simulink model "robust_tracking_LQR"  (R2024b)
settings: Solver=VariableStepAuto  StartTime=0.0  StopTime=10.0  RelTol=1e-3
values from neighbouring files (symbols this model uses):
  current2Torque = mot.Kt    [simulation.m]
  denDriv = [Tdrv 1]    [simulation.m]
  denElect = [mot.L Req]    [simulation.m]
  denMech = [J_eq B_eq]    [simulation.m]
  Ki = Kp / Ti    [PID_SCRIPT.m]    (also in PID_controller.m; simulation.m)
  numDriv = [kdrv]    [simulation.m]
  numElect = [1]    [simulation.m]
  numMech = [1]    [simulation.m]
  speed2Voltage = mot.Ke    [simulation.m]
  Tau = 9.4e-3    (= 0.0094)    [StateSpaceScript.m]
undefined symbols (not defined in the file or in its folder): daq, degs2rpm, denBeam, denHPF, drv, gbox, kappa, Nu, numBeam, numHPF, Nx, rads2rpm, rpm2rads, sens, ssc_LQR_aug
settings Model: Creator=Davide Pillon  LastModifiedBy=fede

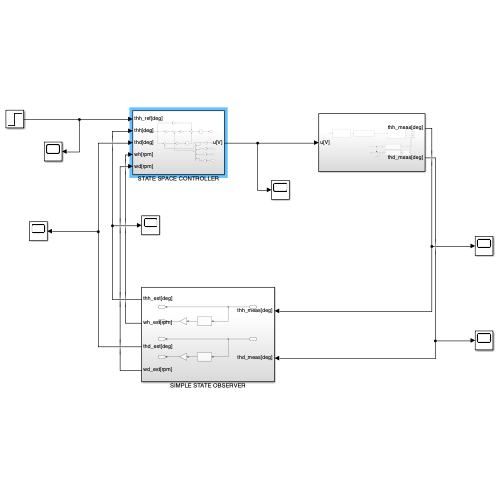
[thumbnail: Simulink's stored preview of the top-level diagram]
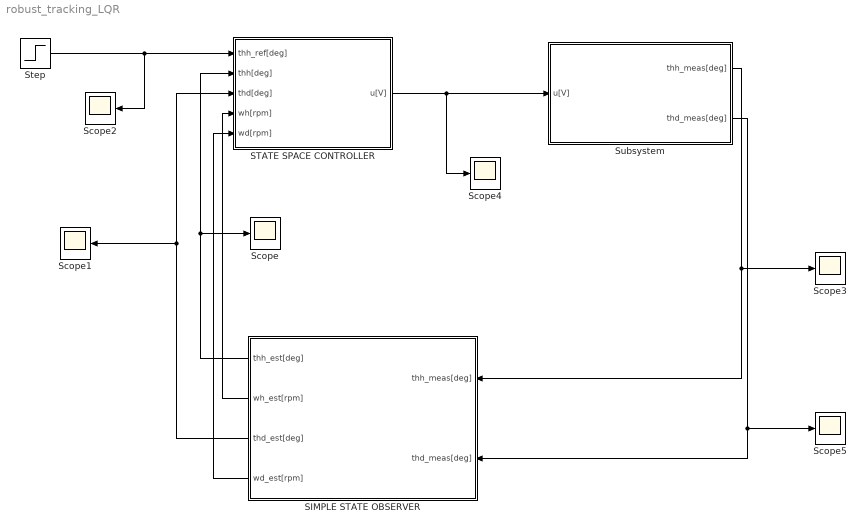
== system robust_tracking_LQR ==
  SIMPLE STATE OBSERVER : Subsystem
  STATE SPACE CONTROLLER : Subsystem
  Scope{,1..5} (6 alike) : Scope
  Step : Step  Time=0  After=50  SampleTime=0
  Subsystem : Subsystem
  wires:
  Step/1 -> STATE SPACE CONTROLLER/1(thh_ref[deg]), Scope2/1
  Subsystem/2(thd_meas[deg]) -> SIMPLE STATE OBSERVER/2(thd_meas[deg]), Scope5/1
  Subsystem/1(thh_meas[deg]) -> SIMPLE STATE OBSERVER/1(thh_meas[deg]), Scope3/1
  SIMPLE STATE OBSERVER/1(thh_est[deg]) -> STATE SPACE CONTROLLER/2(thh[deg]), Scope/1
  SIMPLE STATE OBSERVER/2(wh_est[rpm]) -> STATE SPACE CONTROLLER/4(wh[rpm])
  STATE SPACE CONTROLLER/1(u[V]) -> Scope4/1, Subsystem/1(u[V])
  SIMPLE STATE OBSERVER/4(wd_est[rpm]) -> STATE SPACE CONTROLLER/5(wd[rpm])
  SIMPLE STATE OBSERVER/3(thd_est[deg]) -> STATE SPACE CONTROLLER/3(thd[deg]), Scope1/1

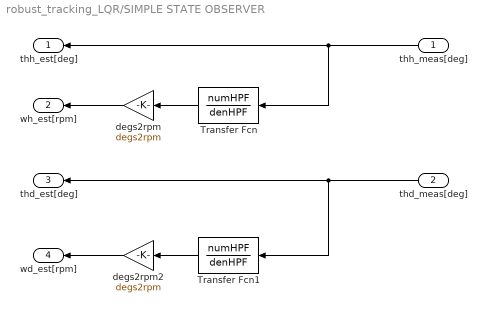
== system robust_tracking_LQR/SIMPLE STATE OBSERVER ==
  thh_meas[deg] : Inport
  thd_meas[deg] : Inport  Port=2
  Transfer Fcn : TransferFcn  Numerator=numHPF  Denominator=denHPF
  Transfer Fcn1 : TransferFcn  Numerator=numHPF  Denominator=denHPF
  degs2rpm : Gain  Gain=degs2rpm
  degs2rpm2 : Gain  Gain=degs2rpm
  thh_est[deg] : Outport
  wh_est[rpm] : Outport  Port=2
  thd_est[deg] : Outport  Port=3
  wd_est[rpm] : Outport  Port=4
  wires:
  Transfer Fcn1/1 -> degs2rpm2/1
  degs2rpm2/1 -> wd_est[rpm]/1
  thd_meas[deg]/1 -> thd_est[deg]/1, Transfer Fcn1/1
  Transfer Fcn/1 -> degs2rpm/1
  degs2rpm/1 -> wh_est[rpm]/1
  thh_meas[deg]/1 -> thh_est[deg]/1, Transfer Fcn/1

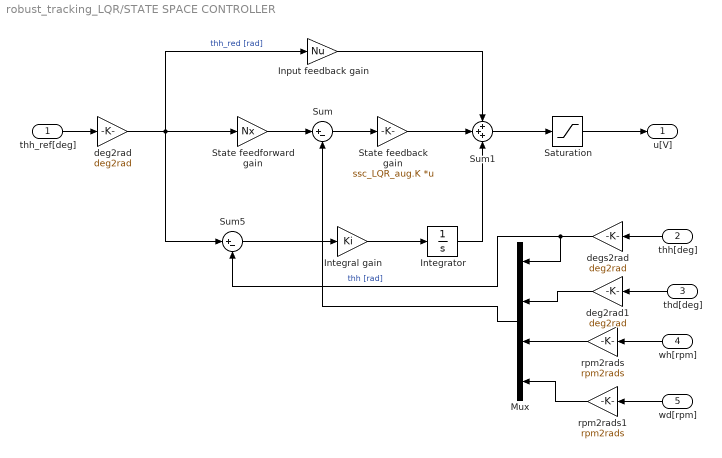
== system robust_tracking_LQR/STATE SPACE CONTROLLER ==
  thh_ref[deg] : Inport
  thh[deg] : Inport  Port=2
  thd[deg] : Inport  Port=3
  wh[rpm] : Inport  Port=4
  wd[rpm] : Inport  Port=5
  Input feedback gain : Gain  Gain=Nu
  Integral gain : Gain  Gain=Ki
  Integrator : Integrator
  Mux : Mux
  Saturation : Saturate  UpperLimit=drv.outmax  LowerLimit=-drv.outmax
  State feedback gain : Gain  Gain=ssc_LQR_aug.K  Multiplication=Matrix(K*u)
  State feedforward gain : Gain  Gain=Nx
  Sum : Sum  Inputs=|+-
  Sum1 : Sum  Inputs=+++
  Sum5 : Sum  Inputs=|+-
  deg2rad : Gain  Gain=deg2rad
  deg2rad1 : Gain  Gain=deg2rad
  degs2rad : Gain  Gain=deg2rad
  rpm2rads : Gain  Gain=rpm2rads
  rpm2rads1 : Gain  Gain=rpm2rads
  u[V] : Outport
  wires:
  Sum/1 -> State feedback gain/1
  Input feedback gain/1 -> Sum1/1
  rpm2rads1/1 -> Mux/4
  Mux/1 -> Sum/2
  Sum1/1 -> Saturation/1
  State feedback gain/1 -> Sum1/2
  thh_ref[deg]/1 -> deg2rad/1
  thd[deg]/1 -> deg2rad1/1
  wh[rpm]/1 -> rpm2rads/1
  Saturation/1 -> u[V]/1
  State feedforward gain/1 -> Sum/1
  rpm2rads/1 -> Mux/3
  deg2rad/1 -> Sum5/1, State feedforward gain/1, Input feedback gain/1  "thh_red [rad]"
  thh[deg]/1 -> degs2rad/1
  deg2rad1/1 -> Mux/2
  wd[rpm]/1 -> rpm2rads1/1
  degs2rad/1 -> Sum5/2, Mux/1  "thh [rad]"
  Sum5/1 -> Integral gain/1
  Integrator/1 -> Sum1/3
  Integral gain/1 -> Integrator/1

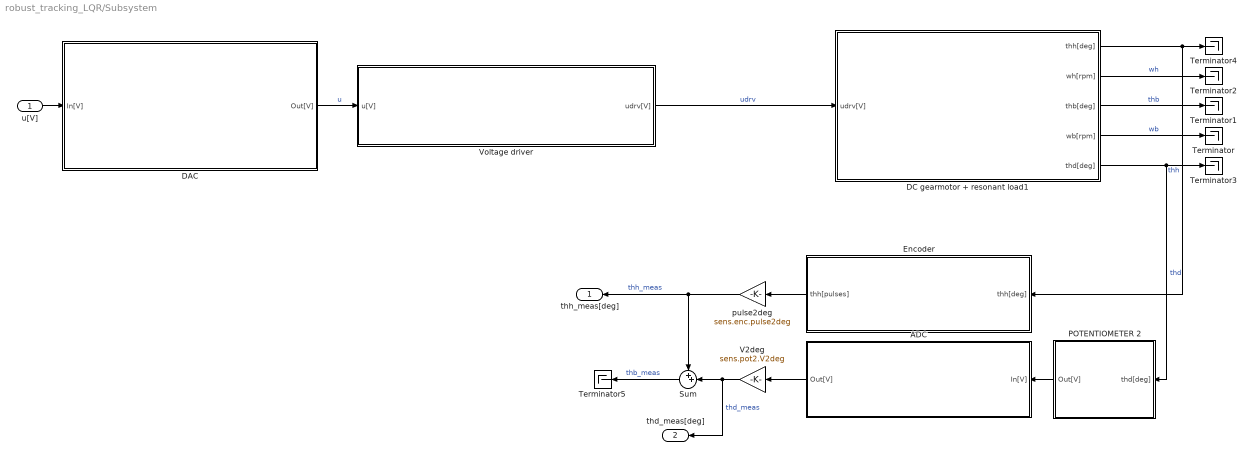
== system robust_tracking_LQR/Subsystem ==
  u[V] : Inport
  ADC : Subsystem
  DAC : Subsystem
  DC gearmotor + resonant load1 : Subsystem
  Encoder : Subsystem
  POTENTIOMETER 2 : Subsystem
  Sum : Sum  Inputs=++|
  Terminator{,1..5} (6 alike) : Terminator
  V2deg : Gain  Gain=sens.pot2.V2deg
  Voltage driver : Subsystem
  pulse2deg : Gain  Gain=sens.enc.pulse2deg
  thh_meas[deg] : Outport
  thd_meas[deg] : Outport  Port=2
  wires:
  DC gearmotor + resonant load1/3(thb[deg]) -> Terminator1/1  "thb"
  DC gearmotor + resonant load1/2(wh[rpm]) -> Terminator2/1  "wh"
  DAC/1(Out[V]) -> Voltage driver/1(u[V])  "u"
  Sum/1 -> Terminator5/1  "thb_meas"
  ADC/1(Out[V]) -> V2deg/1
  DC gearmotor + resonant load1/1(thh[deg]) -> Encoder/1(thh[deg]), Terminator4/1  "thh"
  pulse2deg/1 -> thh_meas[deg]/1, Sum/1  "thh_meas"
  V2deg/1 -> thd_meas[deg]/1, Sum/2  "thd_meas"
  Encoder/1(thh[pulses]) -> pulse2deg/1
  POTENTIOMETER 2/1(Out[V]) -> ADC/1(In[V])
  Voltage driver/1(udrv[V]) -> DC gearmotor + resonant load1/1(udrv[V])  "udrv"
  u[V]/1 -> DAC/1(In[V])
  DC gearmotor + resonant load1/4(wb[rpm]) -> Terminator/1  "wb"
  DC gearmotor + resonant load1/5(thd[deg]) -> POTENTIOMETER 2/1(thd[deg]), Terminator3/1  "thd"

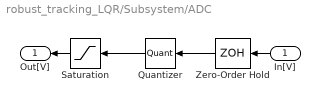
== system robust_tracking_LQR/Subsystem/ADC ==
  In[V] : Inport
  Quantizer : Quantizer  QuantizationInterval=daq.adc.q
  Saturation : Saturate  UpperLimit=daq.adc.fs  LowerLimit=-daq.adc.fs
  Zero-Order Hold : ZeroOrderHold  SampleTime=daq.adc.ts
  Out[V] : Outport
  wires:
  Saturation/1 -> Out[V]/1
  In[V]/1 -> Zero-Order Hold/1
  Zero-Order Hold/1 -> Quantizer/1
  Quantizer/1 -> Saturation/1

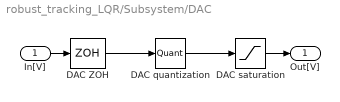
== system robust_tracking_LQR/Subsystem/DAC ==
  In[V] : Inport
  DAC ZOH : ZeroOrderHold  SampleTime=daq.dac.ts
  DAC quantization : Quantizer  QuantizationInterval=daq.dac.q
  DAC saturation : Saturate  UpperLimit=daq.dac.fs  LowerLimit=-daq.dac.fs
  Out[V] : Outport
  wires:
  DAC saturation/1 -> Out[V]/1
  In[V]/1 -> DAC ZOH/1
  DAC ZOH/1 -> DAC quantization/1
  DAC quantization/1 -> DAC saturation/1

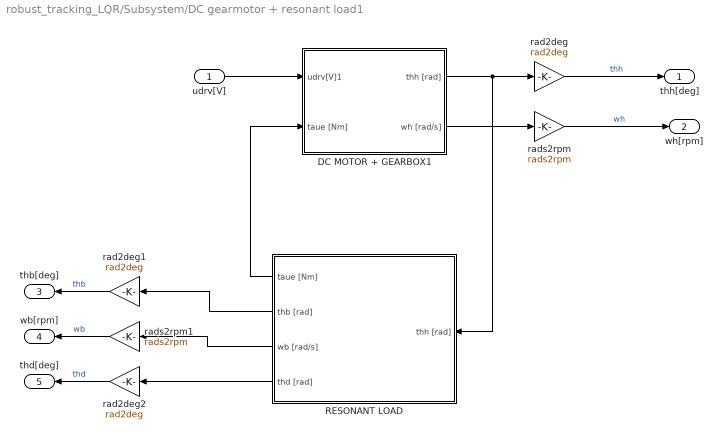
== system robust_tracking_LQR/Subsystem/DC gearmotor + resonant load1 ==
  udrv[V] : Inport
  DC MOTOR + GEARBOX1 : Subsystem
  RESONANT LOAD : Subsystem
  rad2deg : Gain  Gain=rad2deg
  rad2deg1 : Gain  Gain=rad2deg
  rad2deg2 : Gain  Gain=rad2deg
  rads2rpm : Gain  Gain=rads2rpm
  rads2rpm1 : Gain  Gain=rads2rpm
  thh[deg] : Outport
  wh[rpm] : Outport  Port=2
  thb[deg] : Outport  Port=3
  wb[rpm] : Outport  Port=4
  thd[deg] : Outport  Port=5
  wires:
  rad2deg/1 -> thh[deg]/1  "thh"
  rad2deg2/1 -> thd[deg]/1  "thd"
  udrv[V]/1 -> DC MOTOR + GEARBOX1/1(udrv[V]1)
  RESONANT LOAD/4(thd [rad]) -> rad2deg2/1
  RESONANT LOAD/2(thb [rad]) -> rad2deg1/1
  RESONANT LOAD/3(wb [rad/s]) -> rads2rpm1/1
  DC MOTOR + GEARBOX1/2(wh [rad/s]) -> rads2rpm/1
  rad2deg1/1 -> thb[deg]/1  "thb"
  DC MOTOR + GEARBOX1/1(thh [rad]) -> RESONANT LOAD/1(thh [rad]), rad2deg/1
  rads2rpm1/1 -> wb[rpm]/1  "wb"
  RESONANT LOAD/1(taue [Nm]) -> DC MOTOR + GEARBOX1/2(taue [Nm])
  rads2rpm/1 -> wh[rpm]/1  "wh"

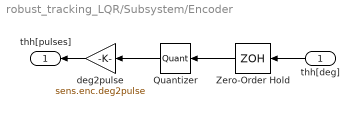
== system robust_tracking_LQR/Subsystem/Encoder ==
  thh[deg] : Inport
  Quantizer : Quantizer  QuantizationInterval=daq.adc.q
  Zero-Order Hold : ZeroOrderHold  SampleTime=daq.adc.ts
  deg2pulse : Gain  Gain=sens.enc.deg2pulse
  thh[pulses] : Outport
  wires:
  thh[deg]/1 -> Zero-Order Hold/1
  deg2pulse/1 -> thh[pulses]/1
  Quantizer/1 -> deg2pulse/1
  Zero-Order Hold/1 -> Quantizer/1

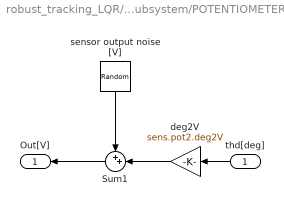
== system robust_tracking_LQR/Subsystem/POTENTIOMETER 2 ==
  thd[deg] : Inport
  Sum1 : Sum  Inputs=++|
  deg2V : Gain  Gain=sens.pot2.deg2V
  sensor output noise [V] : RandomNumber  Variance=sens.pot2.noise.var  SampleTime=sens.pot2.Ts
  Out[V] : Outport
  wires:
  thd[deg]/1 -> deg2V/1
  deg2V/1 -> Sum1/2
  sensor output noise [V]/1 -> Sum1/1
  Sum1/1 -> Out[V]/1

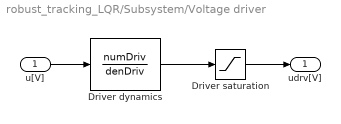
== system robust_tracking_LQR/Subsystem/Voltage driver ==
  u[V] : Inport
  Driver dynamics : TransferFcn  Numerator=numDriv  Denominator=denDriv
  Driver saturation : Saturate  UpperLimit=drv.outmax  LowerLimit=-drv.outmax
  udrv[V] : Outport
  wires:
  u[V]/1 -> Driver dynamics/1
  Driver saturation/1 -> udrv[V]/1
  Driver dynamics/1 -> Driver saturation/1

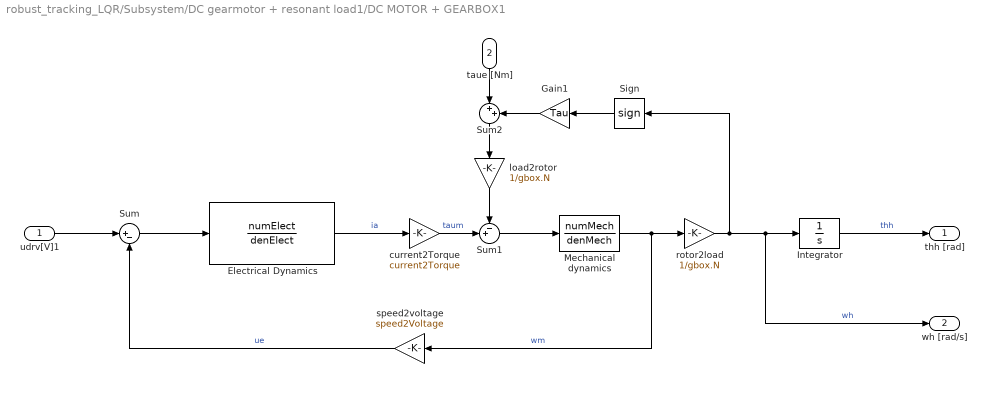
== system robust_tracking_LQR/Subsystem/DC gearmotor + resonant load1/DC MOTOR + GEARBOX1 ==
  udrv[V]1 : Inport
  taue [Nm] : Inport  Port=2
  " Electrical Dynamics" : TransferFcn  Numerator=numElect  Denominator=denElect
  Gain1 : Gain  Gain=Tau
  Integrator : Integrator
  Mechanical dynamics : TransferFcn  Numerator=numMech  Denominator=denMech
  Sign : Signum  ZeroCross=off
  Sum : Sum  Inputs=|+-
  Sum1 : Sum  Inputs=-+|
  Sum2 : Sum  Inputs=|++
  current2Torque : Gain  Gain=current2Torque
  load2rotor : Gain  Gain=1/gbox.N
  rotor2load : Gain  Gain=1/gbox.N
  speed2voltage : Gain  Gain=speed2Voltage
  thh [rad] : Outport
  wh [rad/s] : Outport  Port=2
  wires:
  Integrator/1 -> thh [rad]/1  "thh"
  rotor2load/1 -> Sign/1, wh [rad/s]/1, Integrator/1  "wh"
  udrv[V]1/1 -> Sum/1
  Sum/1 -> " Electrical Dynamics"/1
  current2Torque/1 -> Sum1/2  "taum"
  Sign/1 -> Gain1/1
  Sum2/1 -> load2rotor/1
  speed2voltage/1 -> Sum/2  "ue"
  Gain1/1 -> Sum2/2
  " Electrical Dynamics"/1 -> current2Torque/1  "ia"
  Sum1/1 -> Mechanical dynamics/1
  taue [Nm]/1 -> Sum2/1
  load2rotor/1 -> Sum1/1
  Mechanical dynamics/1 -> speed2voltage/1, rotor2load/1  "wm"

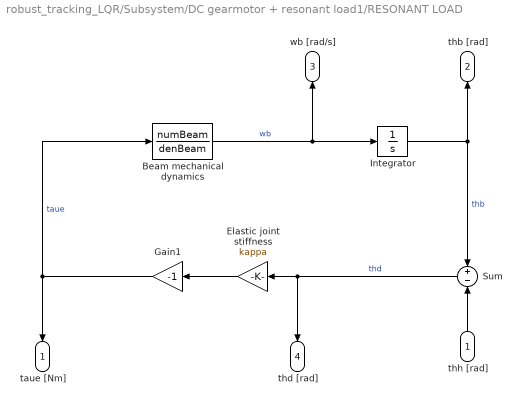
== system robust_tracking_LQR/Subsystem/DC gearmotor + resonant load1/RESONANT LOAD ==
  thh [rad] : Inport
  Beam mechanical dynamics : TransferFcn  Numerator=numBeam  Denominator=denBeam
  Elastic joint stiffness : Gain  Gain=kappa
  Gain1 : Gain  Gain=-1
  Integrator : Integrator
  Sum : Sum  Inputs=+-
  taue [Nm] : Outport
  thb [rad] : Outport  Port=2
  wb [rad/s] : Outport  Port=3
  thd [rad] : Outport  Port=4
  wires:
  Integrator/1 -> thb [rad]/1, Sum/1  "thb"
  Beam mechanical dynamics/1 -> wb [rad/s]/1, Integrator/1  "wb"
  Elastic joint stiffness/1 -> Gain1/1
  Sum/1 -> thd [rad]/1, Elastic joint stiffness/1  "thd"
  Gain1/1 -> taue [Nm]/1, Beam mechanical dynamics/1  "taue"
  thh [rad]/1 -> Sum/2
